simulink model "model_math"  (R2019a)
settings: Solver=FixedStepAuto  StartTime=0.0  StopTime=10.0  FixedStep=0.01  RelTol=1e-3
undefined symbols (not defined in the file): K1
settings Model: Creator=chute  LastModifiedBy=chute
settings DataIOCC: ReturnWorkspaceOutputs=off

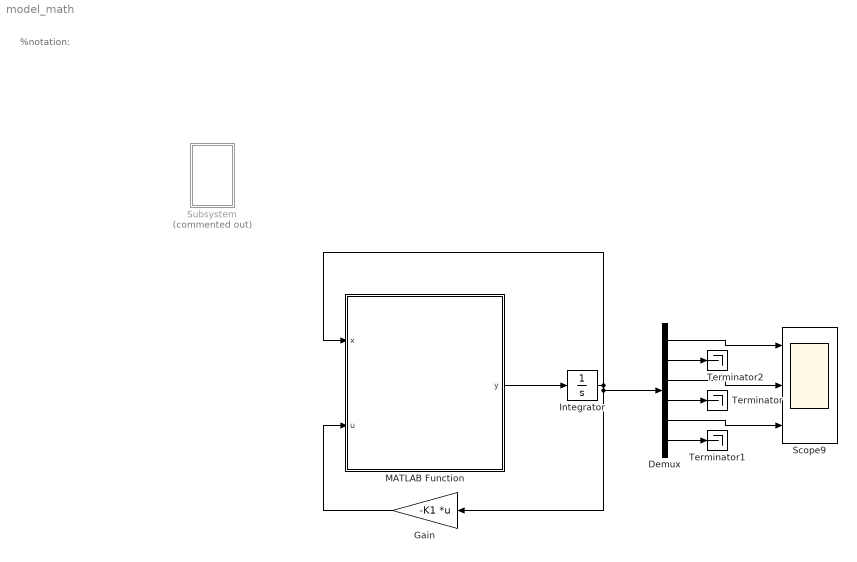
== system model_math ==
  note: %notation:
  Demux : Demux  Outputs=6
  Gain : Gain  Gain=-K1  Multiplication=Matrix(K*u)
  Integrator : Integrator  InitialCondition=[0.01;0.01;0.3;0.01;0.01;0.01]
  MATLAB Function : MATLAB Function  TreatAsAtomicUnit=on
  Scope9 : Scope  NumInputPorts=3
  Subsystem : Subsystem  Commented=on
  Terminator : Terminator
  Terminator1 : Terminator
  Terminator2 : Terminator
  wires:
  Integrator/1 -> Demux/1, Gain/1, MATLAB Function/1(x)
  MATLAB Function/1(y) -> Integrator/1
  Gain/1 -> MATLAB Function/2(u)
  Demux/4 -> Terminator/1
  Demux/2 -> Terminator2/1
  Demux/6 -> Terminator1/1
  Demux/1 -> Scope9/1
  Demux/3 -> Scope9/2
  Demux/5 -> Scope9/3

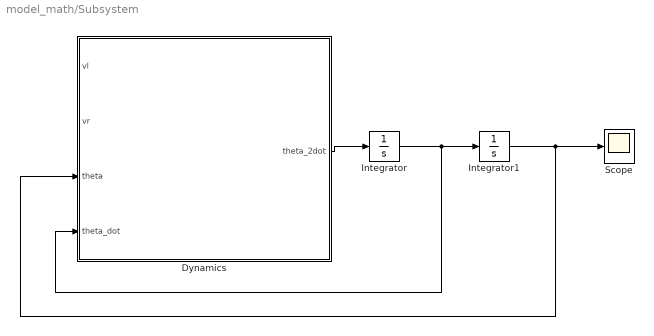
== system model_math/Subsystem ==
  Dynamics : MATLAB Function  TreatAsAtomicUnit=on
  Integrator : Integrator  InitialCondition=[0;0;0]
  Integrator1 : Integrator  InitialCondition=[0;0;0]
  Scope : Scope
  wires:
  Integrator/1 -> Integrator1/1, Dynamics/4(theta_dot)
  Integrator1/1 -> Dynamics/3(theta), Scope/1
  Dynamics/1(theta_2dot) -> Integrator/1

== matlab function model_math/Subsystem/Dynamics ==
  data: vl input; vr input; theta_2dot output; theta input; theta_dot input
function theta_2dot= fcn(vl,vr,theta,theta_dot)
%% declare the paratheta_2dotmeter
g =9.81; % gravity acceleration
m =0.03; % wheel weight
R =0.04; % Wheel radius
M =0.6;  % body weight
W =0.14; % Body width
D =0.04; % Body depth
H =0.144;% Body Height
L =0.144/2;% distance
J_psi  = M*L^2/3; % Body inertia moment
Jw = m*R^2/2;  %Wheel inertia moment
J_phi = M*(W^2+D^2)/12; % Body yaw inertia moment
Jm = 0.00001; % Dc motor inertia moment

n =1 ; %gear ratio
fm = 0.0022; % friction cof between body and DC motor.
fw = 0; % friction cof between wheel and floor
anp = n*Kt/Rm;
bet = n*Kt*Kb/Rm +fm;


the = theta(1);
psi = theta(2);
phi = theta(3);

the_dot = theta_dot(1);
psi_dot = theta_dot(2);
phi_dot = theta_dot(3);


F_the = anp*(vl+vr)-2*(bet+fw)*the_dot+2*bet*psi_dot;
F_psi = -anp*(vl+vr)+2*bet*the_dot-2*bet*psi_dot;
F_phi = W*anp*(vr-vl)/(2*R)-W^2*((bet+fw)*phi_dot)/2*R^2;
tor =[F_the;F_psi;F_phi];

M1 = ...
[2*Jw + 2*Jm*n^2 + R^2*(M + 2*m),  L*M*R*cos(psi)-2*Jm*n^2,          0;
       L*M*R*cos(psi) - 2*Jm*n^2, J_psi + L^2*M + 2*Jm*n^2,          0;
 0,0,J_phi + (W^2*m)/2 + L^2*M*sin(psi)^2 + (W^2*(Jw + Jm*n^2))/(2*R^2)];


C = ...
[0,-L*M*R*psi_dot*sin(psi),0;
 0,0,-L^2*M*phi_dot*cos(psi)*sin(psi);
 0,L^2*M*phi_dot*cos(psi)*sin(psi),L^2*M*psi_dot*cos(psi)*sin(psi)];


G=...
[0;
 -L*M*g*sin(psi);
 0];
dei = transpose([the_dot  psi_dot  phi_dot]);

theta_2dot = inv(M1)*(tor-C*dei-G);

== matlab function model_math/MATLAB Function ==
  data: x input; u input; y output
function y = fcn(x,u)

A=[
         0    1.0000         0         0         0         0
         0   -0.0198   45.3824    0.0198         0         0
         0         0         0    1.0000         0         0
         0    0.0043   51.4164   -0.0043         0         0
         0         0         0         0         0    1.0000
         0         0         0         0         0   -0.0239];
B=[     
         0         0
    0.4536    0.4536
         0         0
   -0.0988   -0.0988
         0         0
   -0.2022    0.2022];
y = A*x+B*u;
